simulink model "Sim3"  (R2014a)
settings: Solver=ode45  StartTime=0.0  StopTime=10.0  RelTol=1e-3
settings Model: Creator=OCAC  LastModifiedBy=OCAC

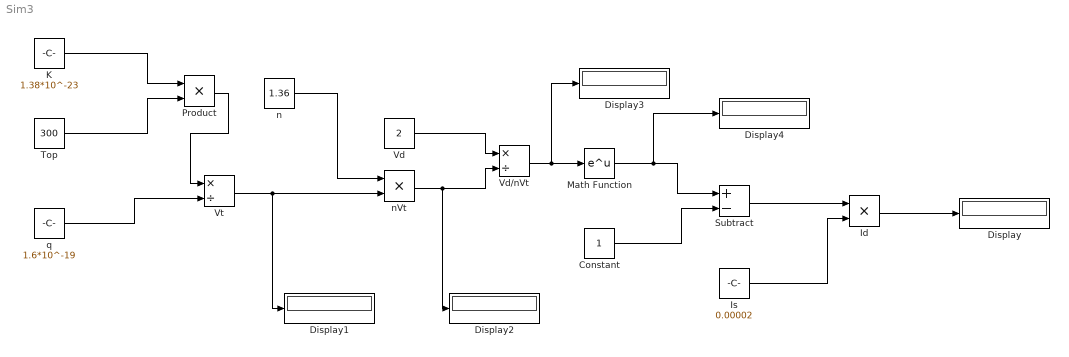
== system Sim3 ==
  Constant : Constant
  Display{,1..4} (5 alike) : Display
  Id : Product
  "Is " : Constant  Value=0.00002
  K : Constant  Value=1.38*10^-23
  Math Function : Math  SaturateOnIntegerOverflow=on
  Product : Product
  Subtract : Sum  Inputs=+-
  Top : Constant  Value=300
  Vd : Constant  Value=2
  Vd/nVt : Product  Inputs=*/
  Vt : Product  Inputs=*/
  n : Constant  Value=1.36
  nVt : Product
  q : Constant  Value=1.6*10^-19
  wires:
  K/1 -> Product/1
  Top/1 -> Product/2
  Product/1 -> Vt/1
  q/1 -> Vt/2
  Vt/1 -> Display1/1, nVt/2
  n/1 -> nVt/1
  Vd/1 -> Vd/nVt/1
  nVt/1 -> Display2/1, Vd/nVt/2
  Vd/nVt/1 -> Display3/1, Math Function/1
  Math Function/1 -> Display4/1, Subtract/1
  Constant/1 -> Subtract/2
  Subtract/1 -> Id/1
  "Is "/1 -> Id/2
  Id/1 -> Display/1
